simulink subsystem "HEVIPS"  (R2024b)
settings: Solver=VariableStepAuto  StartTime=0.0  StopTime=10.0  RelTol=1e-3
undefined symbols (not defined in the file): PlntHevIpsP2GearRatio
libraries: autolibcoupling x2, autolibsharedcoupling x1
settings Model: ModifiedByFormat=The MathWorks, Inc.  Creator=The MathWorks, Inc.  LastModifiedBy=The MathWorks, Inc.
settings SolverCC: MaxZcPerStep=1
settings DebuggingCC: UnconnectedInputMsg=warning  UnconnectedOutputMsg=warning  UnconnectedLineMsg=warning  SubsystemReferenceDiagnosticForUnitTest=warning
settings ModelReferenceCC: EnableRefExpFcnMdlSchedulingChecks=on
settings RTWCC: GPUComputeCapability=3.5  DLArmComputeVersion=19.05

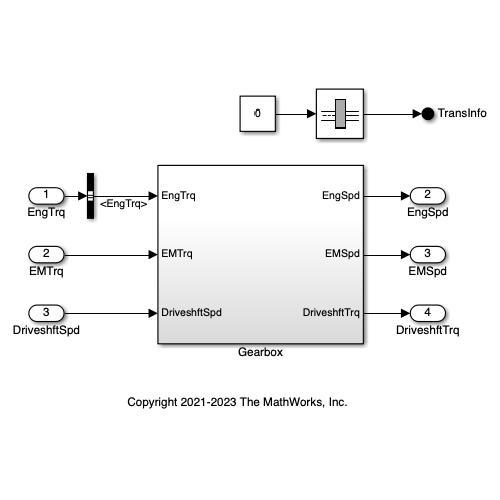
[thumbnail: Simulink's stored preview of the top-level diagram]
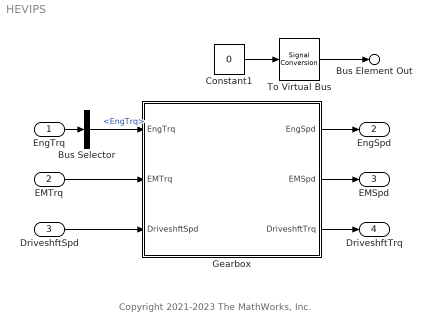
== system HEVIPS ==
  note: Copyright 2021-2023 The MathWorks, Inc.
  EngTrq : Inport
  EMTrq : Inport  Port=2
  DriveshftSpd : Inport  Port=3
  Bus Selector : BusSelector  OutputSignals=EngTrq
  Constant1 : Constant  Value=0  OutDataTypeStr=Bus: TransInfoBUS  SampleTime=Inf
  Gearbox : Subsystem
  To Virtual Bus : SignalConversion  ConversionOutput=Virtual bus  OverrideOpt=off
  Bus Element Out : Outport  PortName=TransInfo
  EngSpd : Outport  Port=2  VectorParamsAs1DForOutWhenUnconnected=off  BusOutputAsStruct=on
  EMSpd : Outport  Port=3  VectorParamsAs1DForOutWhenUnconnected=off  BusOutputAsStruct=on
  DriveshftTrq : Outport  Port=4  VectorParamsAs1DForOutWhenUnconnected=off
  wires:
  EngTrq/1 -> Bus Selector/1
  EMTrq/1 -> Gearbox/2(EMTrq)
  Gearbox/2(EMSpd) -> EMSpd/1
  Gearbox/1(EngSpd) -> EngSpd/1
  Gearbox/3(DriveshftTrq) -> DriveshftTrq/1
  DriveshftSpd/1 -> Gearbox/3(DriveshftSpd)
  To Virtual Bus/1 -> Bus Element Out/1
  Constant1/1 -> To Virtual Bus/1
  Bus Selector/1 -> Gearbox/1(EngTrq)  "<EngTrq>"

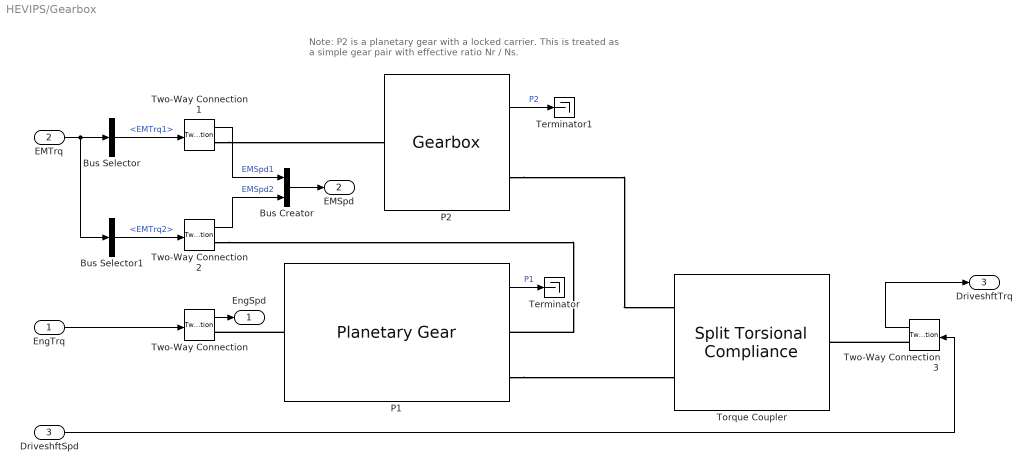
== system HEVIPS/Gearbox ==
  note: Note: P2 is a planetary gear with a locked carrier.
      | This is treated as a simple gear pair with effective ratio Nr / Ns.
  EngTrq : Inport
  EMTrq : Inport  Port=2
  DriveshftSpd : Inport  Port=3
  Bus Creator : BusCreator  Inputs=2
  Bus Selector : BusSelector  OutputSignals=EMTrq1
  Bus Selector1 : BusSelector  OutputSignals=EMTrq2
  P1 : autolibcoupling/Planetary Gear  port_config=Two-way connection  input_config=Torque input - velocity output  Nsp=PlntHevIpsP1SunPlanetRatio  Nsr=PlntHevIpsP1SunRingRatio  Js=PlntHevIpsP1SunInertia  Jp=PlntHevIpsP1PlanetInertia  Jr=PlntHevIpsP1RingInertia  Jc=PlntHevIpsP1CarrInertia  bs=PlntHevIpsP1SunDamp  br=PlntHevIpsP1RingDamp  bp=PlntHevIpsP1PlanetDamp  bc=PlntHevIpsP1CarrDamp  ws_o=PlntHevIpsP1InitSunVel  wc_o=PlntHevIpsP1InitCarrVel  blkID=0
  P2 : autolibcoupling/Gearbox  port_config=Two-way connection  input_config=Torque input - velocity output  DiffEffModelPopup=Constant  InterpMethod=Flat  dirSwitch=on  extTamb=off  N=PlntHevIpsP2GearRatio  J1=PlntHevIpsP2InInertia  J2=PlntHevIpsP2OutInertia  b1=PlntHevIpsP2InDamp  b2=PlntHevIpsP2OutDamp  theta1_o=0  w1_o=PlntHevIpsP2InInitVel  eta=PlntHevIpsP2Eff  eta_tbl=reshape([0.64 0.76 0.8 0.81 0.83 0.84 0.84 0.56 0.73 0.78 0.8 0.83 0.84 0.84 0.54 0.71 0.77 0.8 0.82 0.84 0.84 0.53 0.71 0.77 0.8 0.83 0.84 0.84 0.51 0.71 0.77 0.8 0.83 0.84 0.85 0.52 0.7 0.77 0.8 0.83 0.84 0.85 0.51 0.71 0.76 0.79 0.83 0.84 0.85 0.5 0.69 0.76 0.79 0.82 0.84 0.85 0.45 0.68 0.75 0.78 0.82 0.84 0.85 0.43 0.67 0.74 0.78 0.81 0.83 0.84 0.38 0.63 0.71 0.75 0.8 0.82 0.83 0.81 0.86 0.88 0.89 0.89 0.89 0.9 0.77 0.85 0.87 0.88 0.89 0.9 0.9 0.72 0.82 0.86 0.87 0.88 0.89 0.9 0.68 0.8 0.84 0.86 0.88 0.89 0.89 0.67 0.8 0.84 0.86 0.88 0.89 0.9 0.67 0.8 0.84 0.86 0.88 0.89 0.9 0.65 0.8 0.84 0.86 0.88 0.89 0.9 0.64 0.79 0.83 0.86 0.88 0.89 0.9 0.63 0.78 0.83 0.86 0.88 0.89 0.9 0.59 0.76 0.82 0.85 0.87 0.89 0.9 0.53 0.73 0.8 0.83 0.86 0.88 0.89], 7, 11, 2)  Trq_bpts=[25, 50, 75, 100, 150, 200, 250]  omega_bpts=[52.4 78.5 105 131 157 183 209 262 314 419 524]  Temp_bpts=[290 358]  Tamb=297.15  blkID=0
  Terminator : Terminator
  Terminator1 : Terminator
  Torque Coupler : autolibsharedcoupling/Split Torsional Compliance  port_config=Two-way connection  cplrMode=Shaft merge  extInfo=off  k1=PlntDriveshftStiff  b1=PlntDriveshftDamp  omega1_c=PlntDriveshftDampCutoffFreq  theta1_o=0  domega1_o=0  k2=PlntDriveshftStiff  b2=PlntDriveshftDamp  omega2_c=PlntDriveshftDampCutoffFreq  theta2_o=0  domega2_o=0  blkID=0  aMode=1
      settings: LibrarySourceBlock=autolibcoupling/Split Torsional Compliance
  Two-Way Connection{,1..3} (4 alike) : TwoWayConnection
  EngSpd : Outport  VectorParamsAs1DForOutWhenUnconnected=off
  EMSpd : Outport  Port=2  VectorParamsAs1DForOutWhenUnconnected=off
  DriveshftTrq : Outport  Port=3  VectorParamsAs1DForOutWhenUnconnected=off
  wires:
  Bus Selector/1 -> Two-Way Connection1/1  "<EMTrq1>"
  Bus Creator/1 -> EMSpd/1
  P2/1 -> Terminator1/1  "P2"
  EngTrq/1 -> Two-Way Connection/1
  Two-Way Connection/1 -> EngSpd/1
  Bus Selector1/1 -> Two-Way Connection2/1  "<EMTrq2>"
  P1/1 -> Terminator/1  "P1"
  Two-Way Connection1/1 -> Bus Creator/1  "EMSpd1"
  EMTrq/1 -> Bus Selector/1, Bus Selector1/1
  Two-Way Connection2/1 -> Bus Creator/2  "EMSpd2"
  Two-Way Connection3/1 -> DriveshftTrq/1
  DriveshftSpd/1 -> Two-Way Connection3/1
  connections:
  P1/RConn2 -- Torque Coupler/LConn2
  P1/LConn1 -- Two-Way Connection/RConn1
  Two-Way Connection2/RConn1 -- P1/RConn1
  Two-Way Connection1/RConn1 -- P2/LConn1
  P2/RConn1 -- Torque Coupler/LConn1
  Two-Way Connection3/RConn1 -- Torque Coupler/RConn1
